simulink model "Q5_sim"  (R2021a)
settings: Solver=VariableStepAuto  StartTime=0.0  StopTime=30  RelTol=1e-3
values from neighbouring files (symbols this model uses):
  A = [-1.7,-0.25,0;23,-30,20;0,-200-290,-220-920]    [Q1_code.m]    (also in Q2_code.m; Q3_code.m; Q4_code.m; Q5_code.m)
  BB = [B,B]    [Q5_code.m]
  C = [0,1,0;0,0,1]    [Q1_code.m]    (also in Q2_code.m; Q3_code.m; Q4_code.m; Q5_code.m)
  K = Kba*T    [Q1_code.m]    (also in Q2_code.m = R\B'*P; Q3_code.m = R\B'*P; Q4_code.m = B_s\C_ss; Q5_code.m = R\Bbar'*P)
  L = Lt'    [Q5_code.m]
  x0 = [1;100;200]    [Q1_code.m]    (also in Q2_code.m; Q3_code.m; Q4_code.m; Q5_code.m)
settings Model: Creator=l_w_h  LastModifiedBy=l_w_h

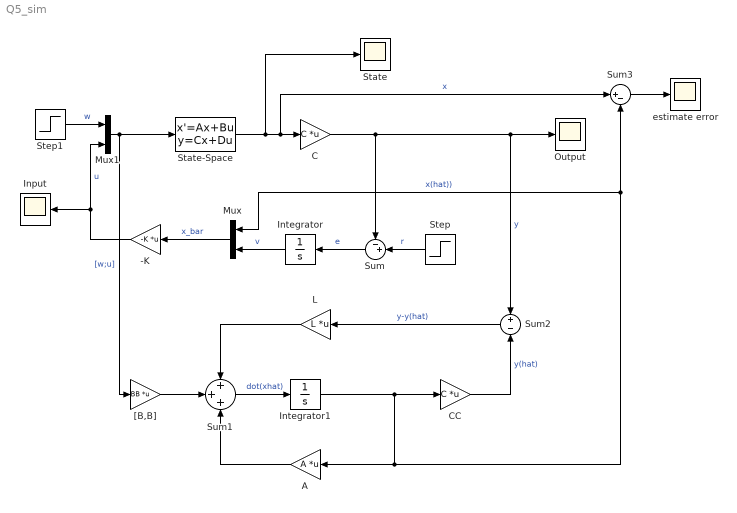
== system Q5_sim ==
  -K : Gain  Gain=-K  Multiplication=Matrix(K*u)
  A : Gain  Gain=A  Multiplication=Matrix(K*u)
  C : Gain  Gain=C  Multiplication=Matrix(K*u)
  CC : Gain  Gain=C  Multiplication=Matrix(K*u)
  Input : Scope
  Integrator : Integrator
  Integrator1 : Integrator
  L : Gain  Gain=L  Multiplication=Matrix(K*u)
  Mux : Mux  Inputs=2
  Mux1 : Mux  Inputs=2
  Output : Scope
  State : Scope
  State-Space : StateSpace  A=A  B=BB  C=eye(3)  D=zeros(3,4)  InitialCondition=x0
  Step : Step  Time=0  After=[100;150]  SampleTime=0
  Step1 : Step  Time=10  After=[-2;5]  SampleTime=0
  Sum : Sum  Inputs=-+|
  Sum1 : Sum  Inputs=+++
  Sum2 : Sum  Inputs=+|-
  Sum3 : Sum  Inputs=|+-
  "[B,B]" : Gain  Gain=BB  Multiplication=Matrix(K*u)
  estimate error : Scope
  wires:
  State-Space/1 -> Sum3/1, C/1, State/1  "x"
  C/1 -> Sum2/1, Output/1, Sum/1  "y"
  Step/1 -> Sum/2  "r"
  Sum/1 -> Integrator/1  "e"
  Integrator/1 -> Mux/2  "v"
  Mux/1 -> -K/1  "x_bar"
  Mux1/1 -> "[B,B]"/1, State-Space/1  "[w;u]"
  -K/1 -> Mux1/2, Input/1  "u"
  Step1/1 -> Mux1/1  "w"
  "[B,B]"/1 -> Sum1/2
  Sum1/1 -> Integrator1/1  "dot(xhat)"
  L/1 -> Sum1/1
  A/1 -> Sum1/3
  Integrator1/1 -> Mux/1, Sum3/2, A/1, CC/1  "x(hat))"
  CC/1 -> Sum2/2  "y(hat)"
  Sum2/1 -> L/1  "y-y(hat)"
  Sum3/1 -> estimate error/1
